simulink model "PIMPID_RO"  (R2013b)
settings: Solver=FixedStepDiscrete  SolverMode=SingleTasking  StartTime=0.0  StopTime=100  FixedStep=0.1  RelTol=1e-3
libraries: xbsIndex_r4 x16
settings Model: Creator=laca  LastModifiedBy=laca

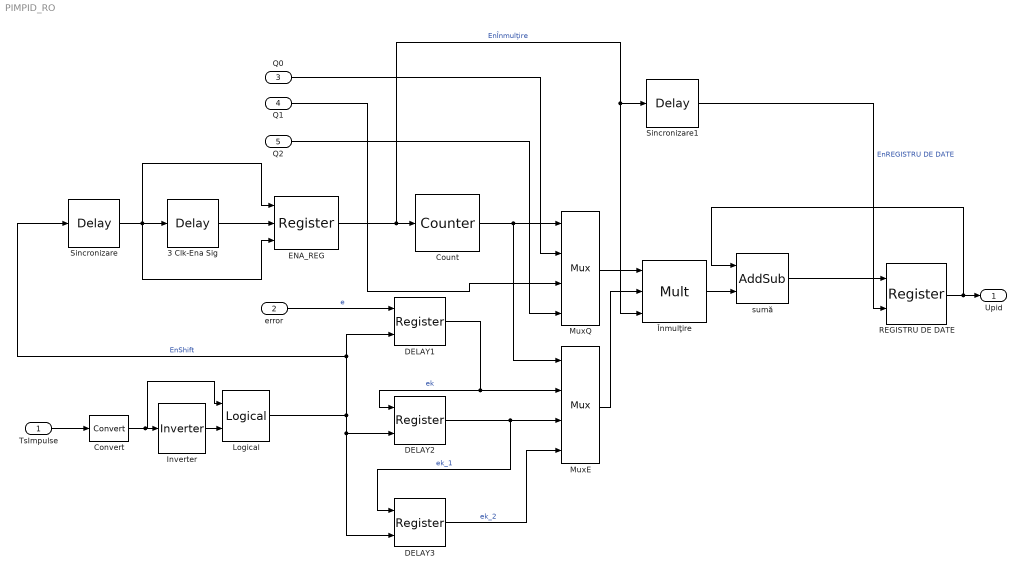
== system PIMPID_RO ==
  TsImpulse : Inport
  error : Inport  Port=2
  Q0 : Inport  Port=3
  Q1 : Inport  Port=4
  Q2 : Inport  Port=5
  3 Clk-Ena Sig : xbsIndex_r4/Delay  rst=off  infoeditControl=Selection of Reset will increase slice count due to use of real FFs and instead of SRLs  en=off  latency=3  dbl_ovrd=off  reg_retiming=off  block_type=delay
  Convert : xbsIndex_r4/Convert  gui_display_data_type=Boolean  arith_type=Boolean  n_bits=16  bin_pt=14  float_type=Single  exp_bits=8  fraction_bits=24  quantization=Truncate  overflow=Wrap  en=off  latency=0  dbl_ovrd=off  pipeline=off  block_type=convert
  Count : xbsIndex_r4/Counter  cnt_type=Count Limited  cnt_to=2  operation=Up  start_count=0  cnt_by_val=1  arith_type=Unsigned  n_bits=2  bin_pt=0  load_pin=off  rst=off  en=on  explicit_period=on  period=1  dbl_ovrd=off  use_behavioral_HDL=off  implementation=Fabric  block_type=counter
      settings: xl_area=[100,0,0,0,0,0,0]
  DELAY1 : xbsIndex_r4/Register  init=0  rst=off  en=on  dbl_ovrd=off  block_type=register
      settings: xl_area=[100,0,0,0,0,0,0]
  DELAY2 : xbsIndex_r4/Register  init=0  rst=off  en=on  dbl_ovrd=off  block_type=register
      settings: xl_area=[100,0,0,0,0,0,0]
  DELAY3 : xbsIndex_r4/Register  init=0  rst=off  en=on  dbl_ovrd=off  block_type=register
  ENA_REG : xbsIndex_r4/Register  init=0  rst=on  en=on  dbl_ovrd=off  block_type=register
  Inverter : xbsIndex_r4/Inverter  en=off  latency=1  dbl_ovrd=off  block_type=inv
  Logical : xbsIndex_r4/Logical  logical_function=AND  inputs=2  en=off  latency=0  precision=Full  arith_type=Unsigned  n_bits=16  bin_pt=0  align_bp=on  dbl_ovrd=off  block_type=logical
  MuxE : xbsIndex_r4/Mux  inputs=3  en=off  latency=0  precision=User Defined  arith_type="Signed  (2's comp)"  n_bits=16  bin_pt=0  quantization=Truncate  overflow=Wrap  dbl_ovrd=off  block_type=mux
      settings: xl_use_area=on  xl_area=[1,0,0,0,0,0,0]
  MuxQ : xbsIndex_r4/Mux  inputs=3  en=off  latency=0  precision=User Defined  arith_type="Signed  (2's comp)"  n_bits=16  bin_pt=0  quantization=Truncate  overflow=Wrap  dbl_ovrd=off  block_type=mux
      settings: xl_area=[1,0,0,0,0,0,0]
  REGISTRU DE DATE : xbsIndex_r4/Register  init=0  rst=off  en=on  dbl_ovrd=off  block_type=register
      settings: xl_area=[100,0,0,0,0,0,0]
  Sincronizare : xbsIndex_r4/Delay  rst=off  infoeditControl=Selection of Reset will increase slice count due to use of real FFs and instead of SRLs  en=off  latency=1  dbl_ovrd=off  reg_retiming=off  block_type=delay
  Sincronizare1 : xbsIndex_r4/Delay  rst=off  infoeditControl=Selection of Reset will increase slice count due to use of real FFs and instead of SRLs  en=off  latency=1  dbl_ovrd=off  reg_retiming=off  block_type=delay
  sumă : xbsIndex_r4/AddSub  mode=Addition  use_carryin=off  use_carryout=off  en=off  latency=0  precision=User Defined  arith_type="Signed  (2's comp)"  n_bits=17  bin_pt=0  quantization=Truncate  overflow=Saturate  dbl_ovrd=off  use_behavioral_HDL=off  hw_selection=Fabric  pipelined=off  block_type=addsub
      settings: xl_area=[100,0,0,0,0,0,0]
  Înmulţire : xbsIndex_r4/Mult  precision=User Defined  arith_type="Signed  (2's comp)"  n_bits=17  bin_pt=0  quantization=Truncate  overflow=Wrap  en=on  latency=1  dbl_ovrd=off  use_behavioral_HDL=off  opt=Area  use_embedded=on  optimum_pipeline=off  pipeline=on  use_rpm=on  placement_style=Triangular  block_type=mult
  Upid : Outport
  wires:
  MuxQ/1 -> Înmulţire/1
  MuxE/1 -> Înmulţire/2
  DELAY2/1 -> DELAY3/1, MuxE/3  "ek_1"
  sumă/1 -> REGISTRU DE DATE/1
  3 Clk-Ena Sig/1 -> ENA_REG/2
  Înmulţire/1 -> sumă/2
  Sincronizare1/1 -> REGISTRU DE DATE/2  "EnREGISTRU DE DATE"
  REGISTRU DE DATE/1 -> Upid/1, sumă/1
  Count/1 -> MuxE/1, MuxQ/1
  ENA_REG/1 -> Sincronizare1/1, Înmulţire/3, Count/1  "EnÎnmulţire"
  Q2/1 -> MuxQ/4
  DELAY3/1 -> MuxE/4  "ek_2"
  Sincronizare/1 -> 3 Clk-Ena Sig/1, ENA_REG/3, ENA_REG/1
  DELAY1/1 -> MuxE/2, DELAY2/1  "ek"
  Q0/1 -> MuxQ/2
  Q1/1 -> MuxQ/3
  Inverter/1 -> Logical/2
  TsImpulse/1 -> Convert/1
  Logical/1 -> DELAY3/2, DELAY2/2, Sincronizare/1, DELAY1/2  "EnShift"
  error/1 -> DELAY1/1  "e"
  Convert/1 -> Inverter/1, Logical/1
